simulink model "financialSolutionsSim"  (R2023a)
settings: Solver=VariableStepAuto  StartTime=0.0  StopTime=10.0  RelTol=1e-3
PreLoadFcn:
  | boiler_simulink=readfis('C:\Users\nagal\OneDrive\Рабочий стол\Boiler.fis');
libraries: fuzblock x1
settings Model: Creator=Jakepps  LastModifiedBy=Jakepps
settings SolverCC: AlgebraicLoopSolver=TrustRegion
settings DataIOCC: LimitDataPoints=on  SaveOutput=off  SaveTime=off
settings OptimizationCC: BlockReduction=off  BooleanDataType=off  LifeSpan=inf
settings DebuggingCC: SaveWithParameterizedLinksMsg=none  UnderspecifiedInitializationDetection=Classic  MergeDetectMultiDrivingBlocksExec=none  SignalResolutionControl=TryResolveAllWithWarning  UnconnectedInputMsg=warning  UnconnectedOutputMsg=warning  UnconnectedLineMsg=warning  AllowSymbolicDim=off  SFUnexpectedBacktrackingDiag=warning  SFNoUnconditionalDefaultTransitionDiag=warning  SFExecutionAtInitializationDiag=none  ArithmeticOperatorsInVariantConditions=warning
settings HardwareCC: TargetUnknown=on
settings ModelReferenceCC: EnableRefExpFcnMdlSchedulingChecks=on
settings SFSimCC: SimUseLocalCustomCode=off  CustomCodeUndefinedFunction=UseInterfaceOnly
settings RTWCC: RTWUseLocalCustomCode=off
settings CodeAppCC: StateflowObjectComments=on
settings GRTTargetCC: TargetLangStandard=C89/C90 (ANSI)

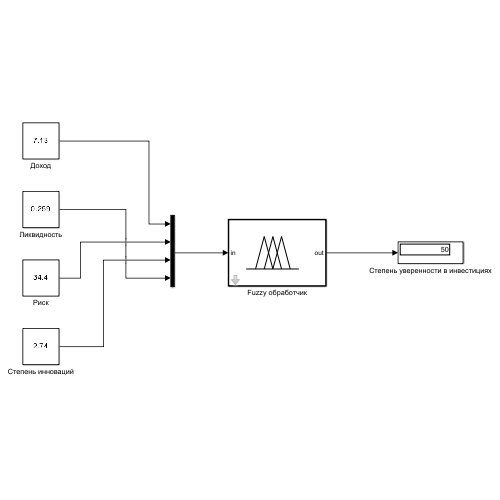
[thumbnail: Simulink's stored preview of the top-level diagram]
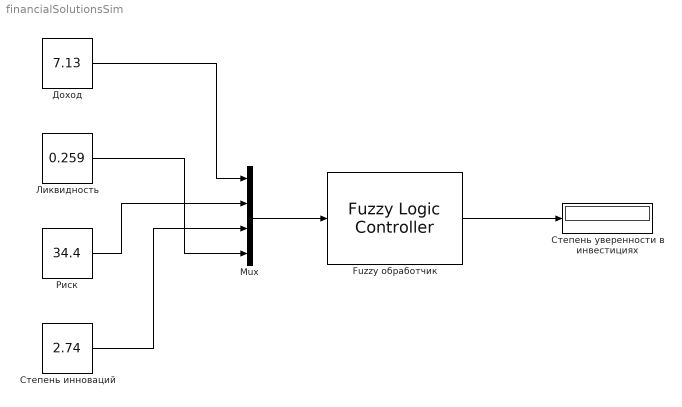
== system financialSolutionsSim ==
  Fuzzy обработчик : fuzblock/Fuzzy Logic  Controller  FIS='C:\Users\nagal\OneDrive\Рабочий стол\Нечеткая\FinancialSolutions.fis'  OutputSampleNumber=101  DataType=double  FuzzifiedInputs=off  RuleFiringStrengths=off  RuleOutputs=off  AggregatedOutputs=off  SimulateUsing=Interpreted execution  OutOfRangeInputValueMessage=warning  NoRuleFiredMessage=warning  EmptyOutputFuzzySetMessage=warning
  Mux : Mux
  Доход : Constant  Value=7.13
  Ликвидность : Constant  Value=0.259
  Риск : Constant  Value=34.4
  Степень инноваций : Constant  Value=2.74
  Степень уверенности в инвестициях : Display
  wires:
  Ликвидность/1 -> Mux/4
  Доход/1 -> Mux/1
  Mux/1 -> Fuzzy обработчик/1
  Fuzzy обработчик/1 -> Степень уверенности в инвестициях/1
  Степень инноваций/1 -> Mux/3
  Риск/1 -> Mux/2
